simulink model "PD_LargeTimeCons"  (R2020b)
settings: Solver=VariableStepAuto  StartTime=0.0  StopTime=50  RelTol=1e-3
undefined symbols (not defined in the file or in its folder): sigbuilder_block
libraries: pid_lib x6
(part 2 of 4)

== matlab function PD_LargeTimeCons/plant/MATLAB Function4 ==
  data: M input; NumTerm input; Thetadd output
function Thetadd = Response(M,NumTerm)
Thetadd=M\NumTerm;
